simulink model "ADRC_SIMU_R1"  (R2018b)
settings: Solver=VariableStepAuto  StartTime=0.0  StopTime=10.0  RelTol=1e-3
settings Model: Creator=Whtest  LastModifiedBy=Whtest

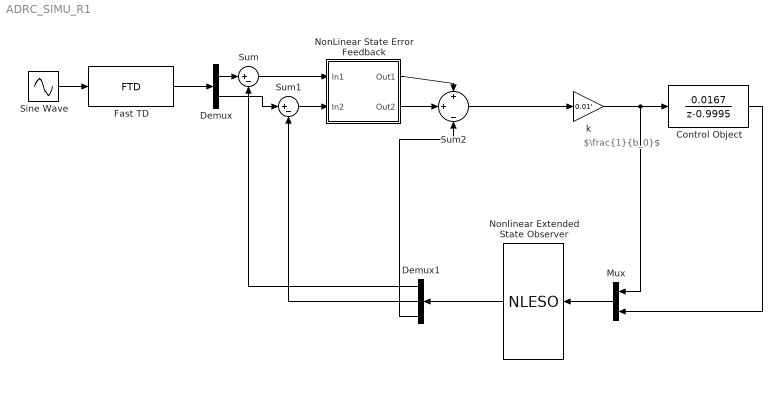
== system ADRC_SIMU_R1 ==
  note: $\frac{1}{b_0}$
  Control Object : DiscreteTransferFcn  Numerator="[ 0    0.0167]"  Denominator="[1.0000   -0.9995]"
  Demux : Demux  Outputs=2
  Demux1 : Demux  Outputs=3
  Fast TD : S-Function  FunctionName=FTD  Parameters=1E-3,1E-2,1000  SFunctionDeploymentMode=off  EnableBusSupport=off
  Mux : Mux  Inputs=2
  NonLinear State Error Feedback : Subsystem
  Nonlinear Extended State Observer : S-Function  FunctionName=NLESO  Parameters=0.1,0.5,10,100,500,50  SFunctionDeploymentMode=off  EnableBusSupport=off
  Sine Wave : Sin  SampleTime=0
  Sum : Sum  Inputs=|+-
  Sum1 : Sum  Inputs=|+-
  Sum2 : Sum  Inputs=+|+|-
  k : Gain  Gain=0.01'
  wires:
  Sine Wave/1 -> Fast TD/1
  Fast TD/1 -> Demux/1
  Demux/1 -> Sum/1
  Demux/2 -> Sum1/1
  Sum/1 -> NonLinear State Error Feedback/1(In1)
  Sum1/1 -> NonLinear State Error Feedback/2(In2)
  Nonlinear Extended State Observer/1 -> Demux1/1
  Demux1/1 -> Sum/2
  Demux1/2 -> Sum1/2
  Demux1/3 -> Sum2/3
  NonLinear State Error Feedback/1(Out1) -> Sum2/1
  NonLinear State Error Feedback/2(Out2) -> Sum2/2
  k/1 -> Mux/1, Control Object/1
  Sum2/1 -> k/1
  Mux/1 -> Nonlinear Extended State Observer/1
  Control Object/1 -> Mux/2

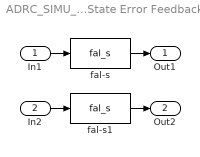
== system ADRC_SIMU_R1/NonLinear State Error Feedback ==
  In1 : Inport
  In2 : Inport  Port=2
  fal-s : S-Function  FunctionName=fal_s  Parameters=.5,0.5  SFunctionDeploymentMode=off  EnableBusSupport=off
  fal-s1 : S-Function  FunctionName=fal_s  Parameters=1,1  SFunctionDeploymentMode=off  EnableBusSupport=off
  Out1 : Outport
  Out2 : Outport  Port=2
  wires:
  In1/1 -> fal-s/1
  In2/1 -> fal-s1/1
  fal-s1/1 -> Out2/1
  fal-s/1 -> Out1/1
